simulink model "SecRwRtStZeroIsPosChk"  (R2018b)
settings: Solver=FixedStepDiscrete  StartTime=0.0  StopTime=10.0  RelTol=1e-3
undefined symbols (not defined in the file or in its folder): KeSMSuSecRwStZeroPosDelta_Val, KeSMSuSecRwStZeroPosTolr_Val
libraries: simulink x3
settings Model: Creator=sn2xws  LastModifiedBy=sn2xws
settings Model: ModifiedHistory=|
  | 2024.7.8 V3.0.0 557模式流程V1.9
  | 2024.8.14 V3.0.1 NotMovFlg 从库函数移出
  | 2024.8.15 V3.0.1 智享模式需要计算目标位置，不能直接判断到位置，posalready赋值0
  | 2024.8.29 V3.0.2 二左的读取信号名改为二右
  | 2024.11.27 V3.0.3 Md57调用时不能直接判断到位置
settings DataIOCC: SaveFormat=StructureWithTime
settings OptimizationCC: DefaultParameterBehavior=Inlined  EnhancedBackFolding=on  PassReuseOutputArgsAs=Individual arguments  ZeroExternalMemoryAtStartup=off  ZeroInternalMemoryAtStartup=off  OptimizeBlockOrder=speed  DifferentSizesBufferReuse=on  OptimizationCustomize=off
settings DebuggingCC: ParameterTunabilityLossMsg=error
settings SFSimCC: MATLABDynamicMemAlloc=off
settings RTWCC: SystemTargetFile=autosar.tlc  GenCodeOnly=on  TemplateMakefile=ert_default_tmf  Description=AUTOSAR  GenerateReport=on  IncludeHyperlinkInReport=on  LaunchReport=on  GenerateTraceInfo=on  GenerateTraceReport=on  GenerateTraceReportSl=on  GenerateTraceReportSf=on  GenerateTraceReportEml=on
settings CodeAppCC: ForceParamTrailComments=on  IgnoreCustomStorageClasses=off  OperatorAnnotations=on  SimulinkDataObjDesc=on  SFDataObjDesc=on  InsertBlockDesc=on
settings STFCustomTargetCC: TargetLangStandard=C99 (ISO)  MultiwordLength=256  ParMdlRefBuildCompliant=on  CompOptLevelCompliant=on  IncludeMdlTerminateFcn=off  CombineOutputUpdateFcns=on  SuppressErrorStatus=on  ERTCustomFileBanners=on  SupportNonFinite=off  SupportComplex=off  SupportContinuousTime=off  SupportNonInlinedSFcns=off  RemoveResetFunc=on  MATLABClassNameForMDSCustomization=Simulink.SoftwareTarget.ERTCustomization  AutosarCompliant=on  UseToolchainInfoCompliant=on  LookupTableObjectStructAxisOrder=2,1,3,4,...  LUTObjectStructOrderEvenSpacing=Size,Table,Breakpoints  SystemTargetFile=autosar.tlc
settings ERTTargetCC: TargetLangStandard=C99 (ISO)  ConcurrentExecutionCompliant=off  IncludeMdlTerminateFcn=off  SuppressErrorStatus=on  SupportNonFinite=off  SupportComplex=off  ModelStepFunctionPrototypeControlCompliant=off  CPPClassGenCompliant=off  AutosarCompliant=on  LookupTableObjectStructAxisOrder=2,1,3,4,...  LUTObjectStructOrderEvenSpacing=Size,Table,Breakpoints  InlinedParameterPlacement=NonHierarchical  ERTCustomFileTemplate=example_file_process.tlc  ERTFilePackagingFormat=Compact

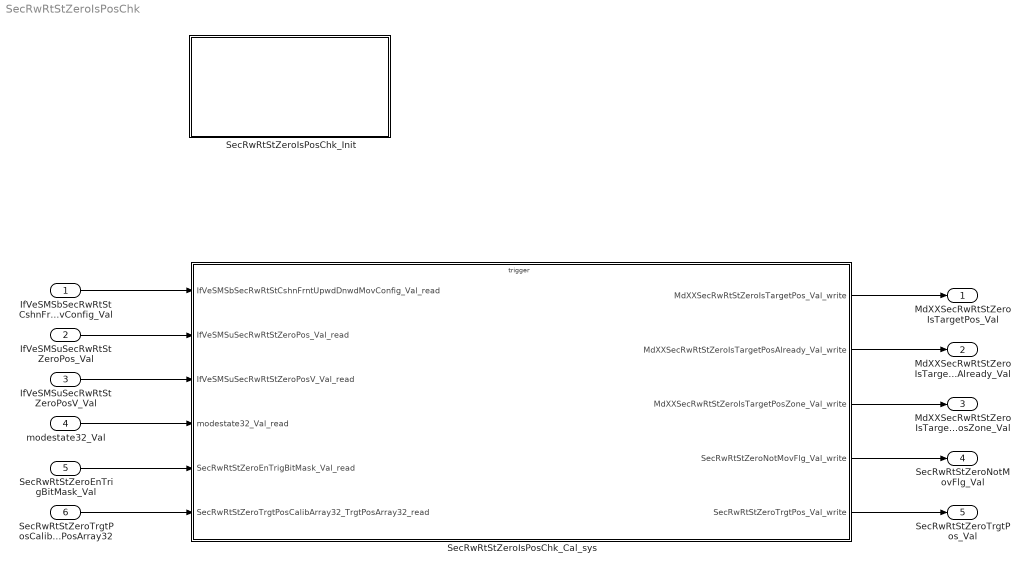
== system SecRwRtStZeroIsPosChk ==
  IfVeSMSbSecRwRtStCshnFrntUpwdDnwdMovConfig_Val : Inport  OutDataTypeStr=boolean  PortDimensions=1
  IfVeSMSuSecRwRtStZeroPos_Val : Inport  Port=2  OutDataTypeStr=uint16  PortDimensions=1
  IfVeSMSuSecRwRtStZeroPosV_Val : Inport  Port=3  OutDataTypeStr=boolean  PortDimensions=1
  modestate32_Val : Inport  Port=4  OutDataTypeStr=uint32  PortDimensions=1
  SecRwRtStZeroEnTrigBitMask_Val : Inport  Port=5  OutDataTypeStr=uint32  PortDimensions=1
  SecRwRtStZeroTrgtPosCalibArray32_TrgtPosArray32 : Inport  Description=|  Port=6  OutDataTypeStr=uint16  PortDimensions=96
      | 0:Pos
      | 1:Max
      | 2:Min
  SecRwRtStZeroIsPosChk_Cal_sys : Subsystem
  SecRwRtStZeroIsPosChk_Init : Subsystem
  MdXXSecRwRtStZeroIsTargetPos_Val : Outport  OutDataTypeStr=uint32  PortDimensions=1
  MdXXSecRwRtStZeroIsTargetPosAlready_Val : Outport  Port=2  OutDataTypeStr=uint32  PortDimensions=1
  MdXXSecRwRtStZeroIsTargetPosZone_Val : Outport  Port=3  OutDataTypeStr=uint32  PortDimensions=1
  SecRwRtStZeroNotMovFlg_Val : Outport  Port=4  OutDataTypeStr=boolean  PortDimensions=1
  SecRwRtStZeroTrgtPos_Val : Outport  Port=5  OutDataTypeStr=uint16  PortDimensions=1
  wires:
  IfVeSMSbSecRwRtStCshnFrntUpwdDnwdMovConfig_Val/1 -> SecRwRtStZeroIsPosChk_Cal_sys/1(IfVeSMSbSecRwRtStCshnFrntUpwdDnwdMovConfig_Val_read)
  IfVeSMSuSecRwRtStZeroPos_Val/1 -> SecRwRtStZeroIsPosChk_Cal_sys/2(IfVeSMSuSecRwRtStZeroPos_Val_read)
  IfVeSMSuSecRwRtStZeroPosV_Val/1 -> SecRwRtStZeroIsPosChk_Cal_sys/3(IfVeSMSuSecRwRtStZeroPosV_Val_read)
  modestate32_Val/1 -> SecRwRtStZeroIsPosChk_Cal_sys/4(modestate32_Val_read)
  SecRwRtStZeroIsPosChk_Cal_sys/1(MdXXSecRwRtStZeroIsTargetPos_Val_write) -> MdXXSecRwRtStZeroIsTargetPos_Val/1
  SecRwRtStZeroIsPosChk_Cal_sys/2(MdXXSecRwRtStZeroIsTargetPosAlready_Val_write) -> MdXXSecRwRtStZeroIsTargetPosAlready_Val/1
  SecRwRtStZeroIsPosChk_Cal_sys/3(MdXXSecRwRtStZeroIsTargetPosZone_Val_write) -> MdXXSecRwRtStZeroIsTargetPosZone_Val/1
  SecRwRtStZeroIsPosChk_Cal_sys/4(SecRwRtStZeroNotMovFlg_Val_write) -> SecRwRtStZeroNotMovFlg_Val/1
  SecRwRtStZeroIsPosChk_Cal_sys/5(SecRwRtStZeroTrgtPos_Val_write) -> SecRwRtStZeroTrgtPos_Val/1
  SecRwRtStZeroEnTrigBitMask_Val/1 -> SecRwRtStZeroIsPosChk_Cal_sys/5(SecRwRtStZeroEnTrigBitMask_Val_read)
  SecRwRtStZeroTrgtPosCalibArray32_TrgtPosArray32/1 -> SecRwRtStZeroIsPosChk_Cal_sys/6(SecRwRtStZeroTrgtPosCalibArray32_TrgtPosArray32_read)

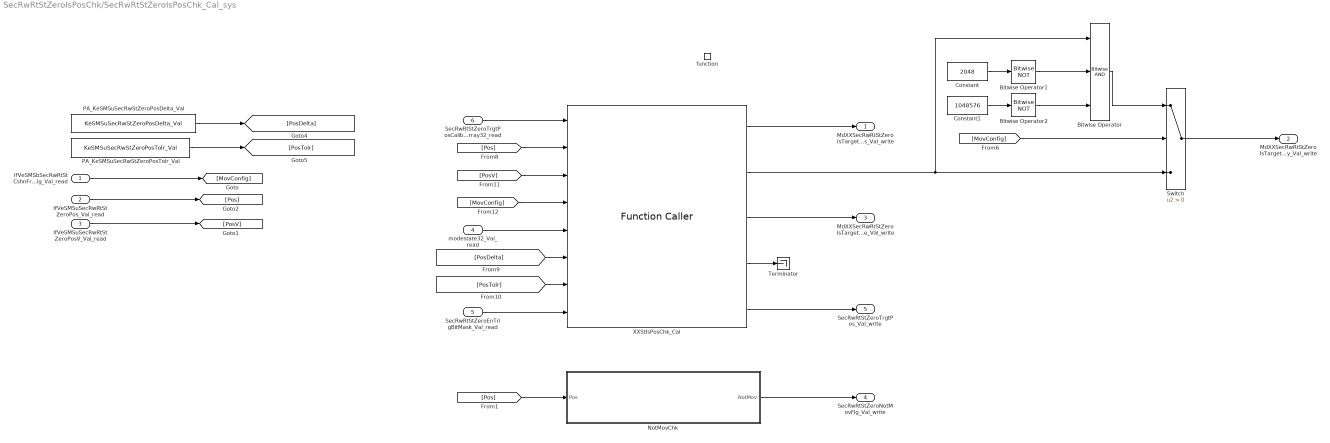
== system SecRwRtStZeroIsPosChk/SecRwRtStZeroIsPosChk_Cal_sys ==
  IfVeSMSbSecRwRtStCshnFrntUpwdDnwdMovConfig_Val_read : Inport
  IfVeSMSuSecRwRtStZeroPos_Val_read : Inport  Port=2
  IfVeSMSuSecRwRtStZeroPosV_Val_read : Inport  Port=3
  modestate32_Val_read : Inport  Port=4
  SecRwRtStZeroEnTrigBitMask_Val_read : Inport  Port=5
  SecRwRtStZeroTrgtPosCalibArray32_TrgtPosArray32_read : Inport  Port=6
  function : TriggerPort  TriggerType=function-call  IsSimulinkFunction=on  FunctionName=SecRwRtStZeroIsPosChk_Cal  VariantControl=(inherit)
  Bitwise Operator : simulink/Logic and Bit Operations/Bitwise Operator  logicop=AND  UseBitMask=off  NumInputPorts=3  BitMask=bin2dec('11011001')  BitMaskRealWorld=Stored Integer
  Bitwise Operator1 : simulink/Logic and Bit Operations/Bitwise Operator  logicop=NOT  UseBitMask=off  BitMask=bin2dec('11011001')  BitMaskRealWorld=Stored Integer
  Bitwise Operator2 : simulink/Logic and Bit Operations/Bitwise Operator  logicop=NOT  UseBitMask=off  BitMask=bin2dec('11011001')  BitMaskRealWorld=Stored Integer
  Constant : Constant  Value=2048  OutDataTypeStr=uint32
  Constant1 : Constant  Value=1048576  OutDataTypeStr=uint32
  NotMovChk : Subsystem
  PA_KeSMSuSecRwStZeroPosDelta_Val : Constant  Value=KeSMSuSecRwStZeroPosDelta_Val
  PA_KeSMSuSecRwStZeroPosTolr_Val : Constant  Value=KeSMSuSecRwStZeroPosTolr_Val
  Switch : Switch  Criteria=u2 > Threshold
  Terminator : Terminator
  XXStIsPosChk_Cal : FunctionCaller  FunctionPrototype=[IsPos,IsPosAlready,IsPosZone,NotMovFlg,StTrgtPos] = XXStIsPosChk_Cal(MdCalibArray32,Pos,PosV,MovConfig,modestate32,PosDelta,PosTolr,StBitMask)  InputArgumentSpecifications=uint16([1;1;1;1;1;1;1;1;1;1;1;1;1;1;1;1;1;1;1;1;1;1;1;1;1;1;1;1;1;1;1;1;1;1;1;1;1;1;1;1;1;1;1;1;1;1;1;1;1;1;1;1;1;1;1;1;1;1;1;1;1;1;1;1;1;1;1;1;1;1;1;1;1;1;1;1;1;1;1;1;1;1;1;1;1;1;1;1;1;1;1;1;1;1;1;1]), uint16(1), boolean(true), boolean(true), uint32(1), uint16(1), uint16(1), uint32(1)  OutputArgumentSpecifications=uint32(1), uint32(1), uint32(1), boolean(true), uint16(1)
  MdXXSecRwRtStZeroIsTargetPos_Val_write : Outport
      settings: EnsureOutportIsVirtual=on
  MdXXSecRwRtStZeroIsTargetPosAlready_Val_write : Outport  Port=2
      settings: EnsureOutportIsVirtual=on
  MdXXSecRwRtStZeroIsTargetPosZone_Val_write : Outport  Port=3
      settings: EnsureOutportIsVirtual=on
  SecRwRtStZeroNotMovFlg_Val_write : Outport  Port=4
      settings: EnsureOutportIsVirtual=on
  SecRwRtStZeroTrgtPos_Val_write : Outport  Port=5
      settings: EnsureOutportIsVirtual=on
  wires:
  PA_KeSMSuSecRwStZeroPosTolr_Val/1 -> [PosTolr]
  PA_KeSMSuSecRwStZeroPosDelta_Val/1 -> [PosDelta]
  XXStIsPosChk_Cal/3 -> MdXXSecRwRtStZeroIsTargetPosZone_Val_write/1
  XXStIsPosChk_Cal/1 -> MdXXSecRwRtStZeroIsTargetPos_Val_write/1
  IfVeSMSbSecRwRtStCshnFrntUpwdDnwdMovConfig_Val_read/1 -> [MovConfig]
  IfVeSMSuSecRwRtStZeroPosV_Val_read/1 -> [PosV]
  IfVeSMSuSecRwRtStZeroPos_Val_read/1 -> [Pos]
  SecRwRtStZeroTrgtPosCalibArray32_TrgtPosArray32_read/1 -> XXStIsPosChk_Cal/1
  modestate32_Val_read/1 -> XXStIsPosChk_Cal/5
  SecRwRtStZeroEnTrigBitMask_Val_read/1 -> XXStIsPosChk_Cal/8
  [Pos] -> XXStIsPosChk_Cal/2
  XXStIsPosChk_Cal/5 -> SecRwRtStZeroTrgtPos_Val_write/1
  [PosV] -> XXStIsPosChk_Cal/3
  [MovConfig] -> XXStIsPosChk_Cal/4
  [PosDelta] -> XXStIsPosChk_Cal/6
  [PosTolr] -> XXStIsPosChk_Cal/7
  [Pos] -> NotMovChk/1(Pos)
  NotMovChk/1(NotMov) -> SecRwRtStZeroNotMovFlg_Val_write/1
  XXStIsPosChk_Cal/4 -> Terminator/1
  Constant/1 -> Bitwise Operator1/1
  XXStIsPosChk_Cal/2 -> Bitwise Operator/1, Switch/3
  Bitwise Operator1/1 -> Bitwise Operator/2
  Bitwise Operator/1 -> Switch/1
  [MovConfig] -> Switch/2
  Switch/1 -> MdXXSecRwRtStZeroIsTargetPosAlready_Val_write/1
  Bitwise Operator2/1 -> Bitwise Operator/3
  Constant1/1 -> Bitwise Operator2/1

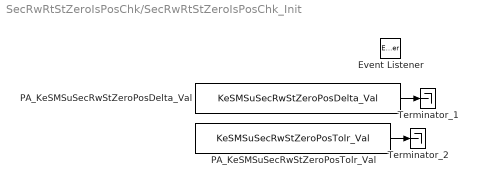
== system SecRwRtStZeroIsPosChk/SecRwRtStZeroIsPosChk_Init ==
  Event Listener : EventListener  EventName=reset
  PA_KeSMSuSecRwStZeroPosDelta_Val : Constant  Value=KeSMSuSecRwStZeroPosDelta_Val
  PA_KeSMSuSecRwStZeroPosTolr_Val : Constant  Value=KeSMSuSecRwStZeroPosTolr_Val
  Terminator_1 : Terminator
  Terminator_2 : Terminator
  wires:
  PA_KeSMSuSecRwStZeroPosDelta_Val/1 -> Terminator_1/1
  PA_KeSMSuSecRwStZeroPosTolr_Val/1 -> Terminator_2/1

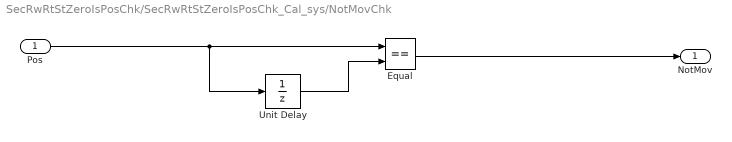
== system SecRwRtStZeroIsPosChk/SecRwRtStZeroIsPosChk_Cal_sys/NotMovChk ==
  Pos : Inport
  Equal : RelationalOperator  Operator===  OutDataTypeStr=boolean  RndMeth=Simplest
  Unit Delay : UnitDelay  SampleTime=-1
  NotMov : Outport
  wires:
  Unit Delay/1 -> Equal/2
  Pos/1 -> Unit Delay/1, Equal/1
  Equal/1 -> NotMov/1
